simulink model "actuator_subsystem"  (R2023b)
settings: Solver=VariableStepAuto  StartTime=0.0  StopTime=10.0  RelTol=1e-3
libraries: autolibbldc x3
settings Model: Creator=tiwan  LastModifiedBy=tiwan

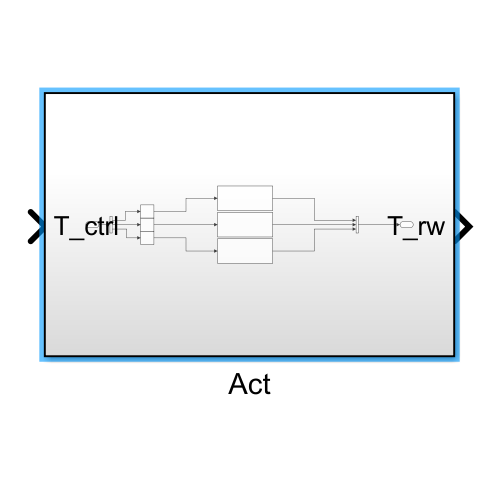
[thumbnail: Simulink's stored preview of the top-level diagram]
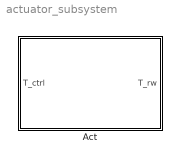
== system actuator_subsystem ==
  Act : Subsystem

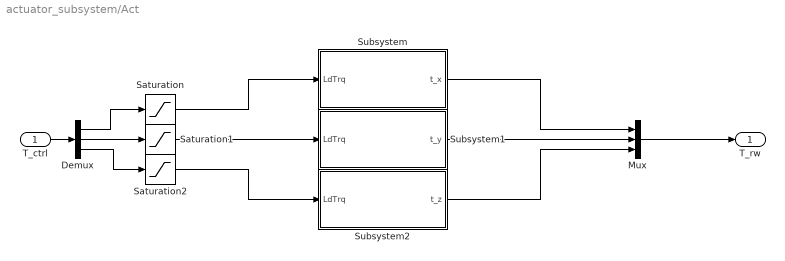
== system actuator_subsystem/Act ==
  T_ctrl : Inport
  Demux : Demux  Outputs=3
  Mux : Mux  Inputs=3
  Saturation : Saturate  UpperLimit=0.2  LowerLimit=-0.2
  Saturation1 : Saturate  UpperLimit=0.2  LowerLimit=-0.2
  Saturation2 : Saturate  UpperLimit=0.2  LowerLimit=-0.2
  Subsystem : Subsystem
  Subsystem1 : Subsystem
  Subsystem2 : Subsystem
  T_rw : Outport
  wires:
  T_ctrl/1 -> Demux/1
  Demux/1 -> Saturation/1
  Demux/2 -> Saturation1/1
  Demux/3 -> Saturation2/1
  Mux/1 -> T_rw/1
  Saturation/1 -> Subsystem/1(LdTrq)
  Saturation1/1 -> Subsystem1/1(LdTrq)
  Saturation2/1 -> Subsystem2/1(LdTrq)
  Subsystem1/1(t_y) -> Mux/2
  Subsystem/1(t_x) -> Mux/1
  Subsystem2/1(t_z) -> Mux/3

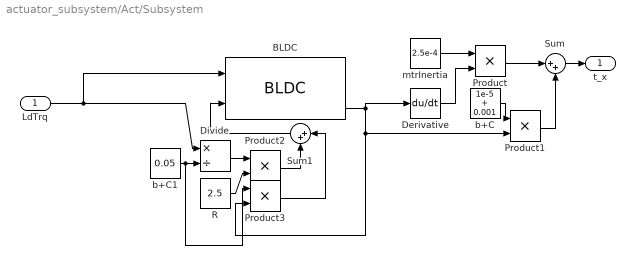
== system actuator_subsystem/Act/Subsystem ==
  LdTrq : Inport
  BLDC : autolibbldc/BLDC  VariantControl=pmsmVariant==pmsmEnum.TorqueInput  MechInput=Torque  SimType=Continuous  BlockSampleTime=25e-6  p=1  Rs=2.5  Ld=0.005  Lq=0.005  Lambda=0.0064  J=2.5e-4  B=2.6369e-06  F=0  Id_init=0  Iq_init=0  Th_init=0  Omega_init=0  RefBlkName='autolibbldc/BLDC'  aMode=5
      settings: LibrarySourceBlock=mcblib/Electrical Systems/Motors/BLDC
  Derivative : Derivative
  Divide : Product  Inputs=*/
  Product{,1..3} (4 alike) : Product
  R : Constant  Value=2.5
  Sum : Sum  Inputs=|++
  Sum1 : Sum  Inputs=|++
  b+C : Constant  Value=1e-5 + 0.001
  b+C1 : Constant  Value=0.05
  mtrInertia : Constant  Value=2.5e-4
  t_x : Outport
  wires:
  Product3/1 -> Sum1/1
  b+C1/1 -> Product3/1, Divide/2
  BLDC/3 -> Product3/2, Product1/2, Derivative/1
  LdTrq/1 -> Divide/1, BLDC/1
  R/1 -> Product2/2
  b+C/1 -> Product1/1
  Derivative/1 -> Product/2
  Sum1/1 -> BLDC/2
  mtrInertia/1 -> Product/1
  Product/1 -> Sum/1
  Divide/1 -> Product2/1
  Product1/1 -> Sum/2
  Product2/1 -> Sum1/2
  Sum/1 -> t_x/1

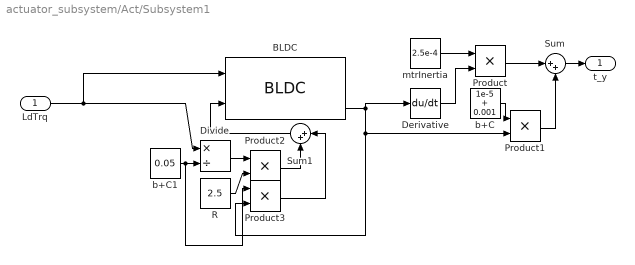
== system actuator_subsystem/Act/Subsystem1 ==
  LdTrq : Inport
  BLDC : autolibbldc/BLDC  VariantControl=pmsmVariant==pmsmEnum.TorqueInput  MechInput=Torque  SimType=Continuous  BlockSampleTime=25e-6  p=1  Rs=2.5  Ld=0.005  Lq=0.005  Lambda=0.0064  J=2.5e-4  B=2.6369e-06  F=0  Id_init=0  Iq_init=0  Th_init=0  Omega_init=0  RefBlkName='autolibbldc/BLDC'  aMode=5
      settings: LibrarySourceBlock=mcblib/Electrical Systems/Motors/BLDC
  Derivative : Derivative
  Divide : Product  Inputs=*/
  Product{,1..3} (4 alike) : Product
  R : Constant  Value=2.5
  Sum : Sum  Inputs=|++
  Sum1 : Sum  Inputs=|++
  b+C : Constant  Value=1e-5 + 0.001
  b+C1 : Constant  Value=0.05
  mtrInertia : Constant  Value=2.5e-4
  t_y : Outport
  wires:
  Product3/1 -> Sum1/1
  b+C1/1 -> Product3/1, Divide/2
  BLDC/3 -> Product3/2, Product1/2, Derivative/1
  LdTrq/1 -> Divide/1, BLDC/1
  R/1 -> Product2/2
  b+C/1 -> Product1/1
  Derivative/1 -> Product/2
  Sum1/1 -> BLDC/2
  mtrInertia/1 -> Product/1
  Product/1 -> Sum/1
  Divide/1 -> Product2/1
  Product1/1 -> Sum/2
  Product2/1 -> Sum1/2
  Sum/1 -> t_y/1

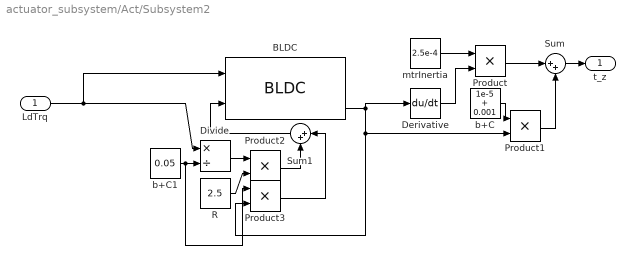
== system actuator_subsystem/Act/Subsystem2 ==
  LdTrq : Inport
  BLDC : autolibbldc/BLDC  VariantControl=pmsmVariant==pmsmEnum.TorqueInput  MechInput=Torque  SimType=Continuous  BlockSampleTime=25e-6  p=1  Rs=2.5  Ld=0.005  Lq=0.005  Lambda=0.0064  J=2.5e-4  B=2.6369e-06  F=0  Id_init=0  Iq_init=0  Th_init=0  Omega_init=0  RefBlkName='autolibbldc/BLDC'  aMode=5
      settings: LibrarySourceBlock=mcblib/Electrical Systems/Motors/BLDC
  Derivative : Derivative
  Divide : Product  Inputs=*/
  Product{,1..3} (4 alike) : Product
  R : Constant  Value=2.5
  Sum : Sum  Inputs=|++
  Sum1 : Sum  Inputs=|++
  b+C : Constant  Value=1e-5 + 0.001
  b+C1 : Constant  Value=0.05
  mtrInertia : Constant  Value=2.5e-4
  t_z : Outport
  wires:
  Product3/1 -> Sum1/1
  b+C1/1 -> Product3/1, Divide/2
  BLDC/3 -> Product3/2, Product1/2, Derivative/1
  LdTrq/1 -> Divide/1, BLDC/1
  R/1 -> Product2/2
  b+C/1 -> Product1/1
  Derivative/1 -> Product/2
  Sum1/1 -> BLDC/2
  mtrInertia/1 -> Product/1
  Product/1 -> Sum/1
  Divide/1 -> Product2/1
  Product1/1 -> Sum/2
  Product2/1 -> Sum1/2
  Sum/1 -> t_z/1
